simulink model "parametrefarkli"  (R2017b)
settings: Solver=VariableStepAuto  StartTime=0.0  StopTime=10.0  RelTol=1e-3
undefined symbols (not defined in the file or in its folder): Ts_Power
libraries: powerlib x65, powerlib_extras x60, powerlib_meascontrol x5, simulink x3, re_lib x3
(part 1 of 3)
settings Model: Creator=ongun  LastModifiedBy=ongun

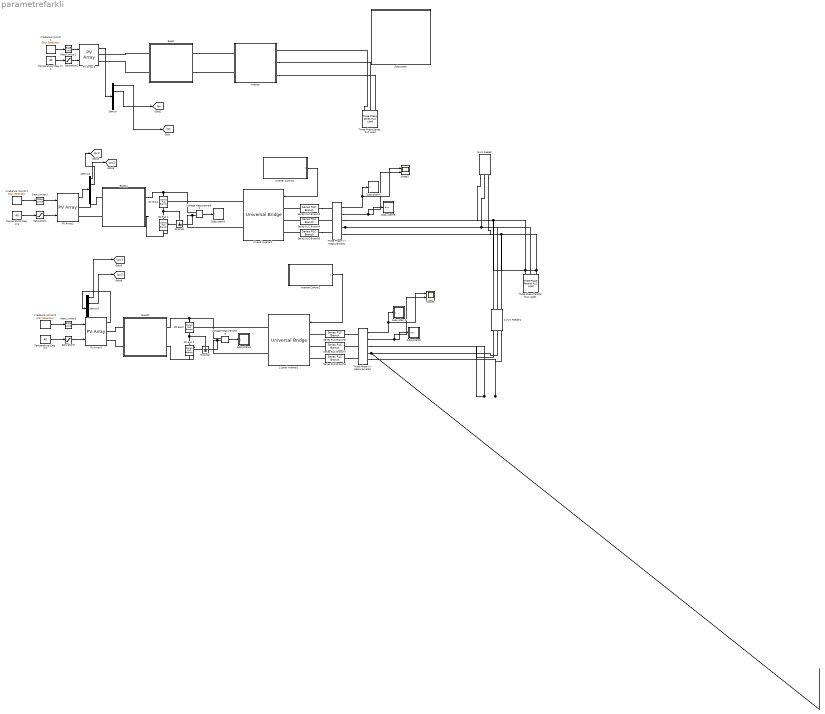
== system parametrefarkli ==
  11-km Feeder1 : powerlib/Elements/Distributed Parameters Line  Phases=3  Frequency=50  Resistance=[0.1153 0.413]  Inductance=[1.05e-3 3.32e-3]  Capacitance=[11.33e-009 5.01e-009]  Length=3  x1=[0 0 0;0 0 0;1.5707963267949 1.5707963267949 1.5707963267949]  x2=[0 0 0;0 0 0;1.5707963267949 1.5707963267949 1.5707963267949]  x3=[0 0 0;0 0 0;1.5707963267949 1.5707963267949 1.5707963267949]  x4=[0 0 0;0 0 0;1.5707963267949 1.5707963267949 1.5707963267949]  x5=1.22351460963897e-05  V1=[0 0 0;0 0 0;1.571 1.571 1.571]  V2=[0 0 0;0 0 0;1.571 1.571 1.571]  I1=[0 0 0;0 0 0;1.571 1.571 1.571]  I2=[0 0 0;0 0 0;1.571 1.571 1.571]  nHarmo=1  Measurements=None
      settings: SourceProductName=Simscape Power Systems
  2 Level Inverter1 : powerlib/Power Electronics/Universal Bridge  Arms=3  SnubberResistance=1e5  SnubberCapacitance=inf  Device=IGBT / Diodes  Ron=1e-3  Lon=0  ForwardVoltages="[  0  0  ]"  ForwardVoltage=0  GTOparameters=[ 10e-6 , 20e-6 ]  IGBTparameters=[ 1e-6 , 2e-6 ]  Measurements=UAB UBC UCA UDC voltages  Measurements_2=None  converterType=Rectifier
  2 Level Inverter2 : powerlib/Power Electronics/Universal Bridge  Arms=3  SnubberResistance=1e5  SnubberCapacitance=inf  Device=IGBT / Diodes  Ron=1e-3  Lon=0  ForwardVoltages="[  0  0  ]"  ForwardVoltage=0  GTOparameters=[ 10e-6 , 20e-6 ]  IGBTparameters=[ 1e-6 , 2e-6 ]  Measurements=UAB UBC UCA UDC voltages  Measurements_2=None  converterType=Rectifier
  8-km Feeder : powerlib/Elements/Distributed Parameters Line  Phases=3  Frequency=50  Resistance=[0.1153 0.413]  Inductance=[1.05e-3 3.32e-3]  Capacitance=[11.33e-009 5.01e-009]  Length=100  x1=[0 0 0;0 0 0;1.5707963267949 1.5707963267949 1.5707963267949]  x2=[0 0 0;0 0 0;1.5707963267949 1.5707963267949 1.5707963267949]  x3=[0 0 0;0 0 0;1.5707963267949 1.5707963267949 1.5707963267949]  x4=[0 0 0;0 0 0;1.5707963267949 1.5707963267949 1.5707963267949]  x5=0.00040783820321299  V1=[0 0 0;0 0 0;1.571 1.571 1.571]  V2=[0 0 0;0 0 0;1.571 1.571 1.571]  I1=[0 0 0;0 0 0;1.571 1.571 1.571]  I2=[0 0 0;0 0 0;1.571 1.571 1.571]  nHarmo=1  Measurements=None
      settings: SourceProductName=Simscape Power Systems
  Boost : Subsystem
      mask Display: disp('Boost Converter')
  Boost1 : Subsystem
      mask Display: disp('Boost Converter')
  Boost2 : Subsystem
      mask Display: disp('Boost Converter')
  DC Bus 1 : powerlib/Elements/Series RLC Branch  LConnTagsString=__new0  RConnTagsString=__new0  BranchType=C  Resistance=1  Inductance=5e-03  SetiL0=off  InitialCurrent=0  Capacitance=10e-3/2  Setx0=off  InitialVoltage=1000/2  Measurements=None
  DC Bus 2 : powerlib/Elements/Series RLC Branch  LConnTagsString=__new0  RConnTagsString=__new0  BranchType=C  Resistance=1  Inductance=5e-03  SetiL0=off  InitialCurrent=0  Capacitance=10e-3/2  Setx0=off  InitialVoltage=1000/2  Measurements=None
  DC Bus1 : powerlib/Elements/Series RLC Branch  LConnTagsString=__new0  RConnTagsString=__new0  BranchType=C  Resistance=1  Inductance=5e-03  SetiL0=off  InitialCurrent=0  Capacitance=10e-3/2  Setx0=off  InitialVoltage=1000/2  Measurements=None
  DC Bus2 : powerlib/Elements/Series RLC Branch  LConnTagsString=__new0  RConnTagsString=__new0  BranchType=C  Resistance=1  Inductance=5e-03  SetiL0=off  InitialCurrent=0  Capacitance=10e-3/2  Setx0=off  InitialVoltage=1000/2  Measurements=None
  Demux : Demux  Outputs=5
  Demux2 : Demux  Outputs=5
  Demux3 : Demux  Outputs=5
  Ground1 : powerlib/Elements/Ground  LConnTagsString=a
  Ground2 : powerlib/Elements/Ground  LConnTagsString=a
  Inverter : Subsystem
      mask Display: disp('DC/AC Inverter')
  Inverter Control1 : Subsystem
  Inverter Control2 : Subsystem
  Irradiance (W/m2) 1 : powerlib_meascontrol/Pulse & Signal Generators/Stair Generator  t=[0, 0.5, 2.3]  e=[1,0.05, 1.0]*1000  Ts=Ts_Power
      settings: SourceProductName=Simscape Power Systems
  Irradiance (W/m2)1 : powerlib_meascontrol/Pulse & Signal Generators/Stair Generator  t=[0, 0.4, 1.0]  e=[1, 0.2, 1]*1000  Ts=5e-5
      settings: SourceProductName=Simscape Power Systems
  Irradiance (W/m2)2 : powerlib_meascontrol/Pulse & Signal Generators/Stair Generator  t=[0, 0.4, 1.0]  e=[1, 0.2, 1]*1000  Ts=5e-5
      settings: SourceProductName=Simscape Power Systems
  PV Array 1 : re_lib/Solar/PV Array  Npar=64  Nser=5  PlotType=array @ 1000 W/m2 & specified temperatures  S_vec="[ 1000  500  100 ]"  Temp_C_vec="[ 45 25  ]"  ModuleName=SunPower SPR-315E-WHT-D  PlotWhenSelected=off  Pm=315.072  Ncell=96  Voc=64.6  Isc=6.14  Vm=54.7  Im=5.76  beta_Voc_pc=-0.27269  alpha_Isc_pc=0.061694  beta_Voc=-0.17616  alpha_Isc=0.003788  IL=6.1461  I0=6.5043e-12  nI=0.9507  Rsh=430.0559  Rs=0.43042  BAL=off  Tc=1e-6  Tfilter=5e-5
  PV Array2 : re_lib/Solar/PV Array  Npar=88  Nser=7  PlotType=array @ 1000 W/m2 & specified temperatures  S_vec="[ 1000  500  100 ]"  Temp_C_vec="[ 45 25  ]"  ModuleName=SunPower SPR-415E-WHT-D  PlotWhenSelected=off  Pm=414.801  Ncell=128  Voc=85.3  Isc=6.09  Vm=72.9  Im=5.69  beta_Voc_pc=-0.229  alpha_Isc_pc=0.030706  beta_Voc=-0.19534  alpha_Isc=0.00187  IL=6.0978  I0=7.1712e-13  nI=0.87223  Rsh=419.7813  Rs=0.5371  BAL=on  Tc=1e-6  Tfilter=5e-5
      settings: AttributesFormatString=|
      | %<ModuleName>
      | %<Nser>-module string
      | %<Npar> parallel strings
  PV Array3 : re_lib/Solar/PV Array  Npar=88  Nser=7  PlotType=array @ 1000 W/m2 & specified temperatures  S_vec="[ 1000  500  100 ]"  Temp_C_vec="[ 45 25  ]"  ModuleName=SunPower SPR-415E-WHT-D  PlotWhenSelected=off  Pm=414.801  Ncell=128  Voc=85.3  Isc=6.09  Vm=72.9  Im=5.69  beta_Voc_pc=-0.229  alpha_Isc_pc=0.030706  beta_Voc=-0.19534  alpha_Isc=0.00187  IL=6.0978  I0=7.1712e-13  nI=0.87223  Rsh=419.7813  Rs=0.5371  BAL=on  Tc=1e-6  Tfilter=5e-5
      settings: AttributesFormatString=|
      | %<ModuleName>
      | %<Nser>-module string
      | %<Npar> parallel strings
  Rate Limiter1 : RateLimiter  RisingSlewLimit=6000  FallingSlewLimit=-6000  SampleTimeMode=inherited  InitialCondition=1000
  Rate Limiter2 : RateLimiter  RisingSlewLimit=8000  FallingSlewLimit=-8000  SampleTimeMode=inherited  InitialCondition=1000
  Rate Limiter3 : RateLimiter  RisingSlewLimit=6000  FallingSlewLimit=-6000  SampleTimeMode=inherited  InitialCondition=1000
  Saturation1 : Saturate  UpperLimit=55  LowerLimit=5
  Saturation2 : Saturate  UpperLimit=55  LowerLimit=5
  Saturation3 : Saturate  UpperLimit=55  LowerLimit=5
  Scope1 : Scope  NumInputPorts=2
  Scope2 : Scope  NumInputPorts=2
  Series RLC Branch{4..9} (6 alike) : powerlib/Elements/Series RLC Branch  LConnTagsString=__new0  RConnTagsString=__new0  BranchType=RL  Resistance=0.1  Inductance=30e-3  SetiL0=off  InitialCurrent=0  Capacitance=1e-6  Setx0=off  InitialVoltage=0  Measurements=Branch voltage
  Subsystem : Subsystem
      mask Display: disp('Measurements')
  Subsystem4 : Subsystem
  Subsystem5 : Subsystem
  Subsystem6 : Subsystem
  Subsystem7 : Subsystem
  Subsystem8 : Subsystem
  Subsystem9 : Subsystem
  Temperature (Deg. C) 1 : Constant  Value=40
  Temperature (Deg. C)1 : Constant  Value=40
  Temperature (Deg. C)2 : Constant  Value=40
  Three-Phase Parallel RLC Load1 : powerlib/Elements/Three-Phase Parallel RLC Load  LConnTagsString=A|B|C  Configuration=Y (grounded)  NominalVoltage=(25000)*1  Vabc=[1e3 1e3 1e3]  Vabcp=[1e3 1e3 1e3]  NominalFrequency=60  UnbalancedPower=off  ActivePower=100e3  InductivePower=0  CapacitivePower=0  Pabc=[10e3 9e3 11e3]  QLabc=[100 90 110]  QCabc=[100 90 110]  Pabcp=[10e3 9e3 11e3]  QLabcp=[100 90 110]  QCabcp=[100 90 110]  Measurements=None  LoadType=constant PQ
  Three-Phase Series RLC Load : powerlib/Elements/Three-Phase Series RLC Load  LConnTagsString=A|B|C  Configuration=Y (grounded)  NominalVoltage=1000  Vabc=[1e3 1e3 1e3]  Vabcp=[1e3 1e3 1e3]  NominalFrequency=60  UnbalancedPower=off  ActivePower=10e3  InductivePower=100  CapacitivePower=100  Pabc=[10e3 9e3 11e3]  QLabc=[100 90 110]  QCabc=[100 90 110]  Pabcp=[10e3 9e3 11e3]  QLabcp=[100 90 110]  QCabcp=[100 90 110]  Measurements=None  LoadType=constant Z
  Three-Phase V-I Measurement1 : powerlib/Measurements/Three-Phase V-I Measurement  VoltageMeasurement=phase-to-ground  SetLabelV=off  LabelV=Vabc  Vpu=off  VpuLL=off  CurrentMeasurement=yes  SetLabelI=off  LabelI=Iabc  Ipu=off  Pbase=100e6  Vbase=500e3  OutputType=Complex  PhasorSimulation=off  PSBequivalent=0
  Three-Phase V-I Measurement2 : powerlib/Measurements/Three-Phase V-I Measurement  VoltageMeasurement=phase-to-ground  SetLabelV=off  LabelV=Vabc  Vpu=off  VpuLL=off  CurrentMeasurement=yes  SetLabelI=off  LabelI=Iabc  Ipu=off  Pbase=100e6  Vbase=500e3  OutputType=Complex  PhasorSimulation=off  PSBequivalent=0
  Voltage Measurement2 : powerlib/Measurements/Voltage Measurement  PhasorSimulation=off  OutputType=Complex  PSBequivalent=0
  Voltage Measurement3 : powerlib/Measurements/Voltage Measurement  PhasorSimulation=off  OutputType=Complex  PSBequivalent=0
  tag scope: Ipv2=global, Ipv3=global, Ipv=global, Vpv2=global, Vpv3=global, Vpv=global
  wires:
  PV Array 1/1 -> Demux/1
  Demux/1 -> [Vpv]
  Demux/2 -> [Ipv]
  Rate Limiter2/1 -> PV Array 1/1
  Temperature (Deg. C) 1/1 -> Saturation2/1
  Saturation2/1 -> PV Array 1/2
  Irradiance (W/m2) 1/1 -> Rate Limiter2/1
  Demux3/1 -> [Vpv3]
  Demux3/2 -> [Ipv3]
  Three-Phase V-I Measurement2/1 -> Scope2/1, Subsystem7/1(Vabc)
  Saturation3/1 -> PV Array3/2
  Inverter Control2/1(S) -> 2 Level Inverter2/1
  Voltage Measurement3/1 -> Subsystem8/1(Vdcinv)
  Three-Phase V-I Measurement2/2 -> Scope2/2, Subsystem9/1(Iabc)
  Temperature (Deg. C)1/1 -> Saturation1/1
  Three-Phase V-I Measurement1/2 -> Scope1/2, Subsystem6/1(Iabc)
  Rate Limiter1/1 -> PV Array2/1
  Voltage Measurement2/1 -> Subsystem5/1(Vdcinv)
  Inverter Control1/1(S) -> 2 Level Inverter1/1
  Three-Phase V-I Measurement1/1 -> Scope1/1, Subsystem4/1(Vabc)
  PV Array2/1 -> Demux2/1
  Irradiance (W/m2)2/1 -> Rate Limiter3/1
  Rate Limiter3/1 -> PV Array3/1
  Saturation1/1 -> PV Array2/2
  PV Array3/1 -> Demux3/1
  Temperature (Deg. C)2/1 -> Saturation3/1
  Irradiance (W/m2)1/1 -> Rate Limiter1/1
  Demux2/2 -> [Ipv2]
  Demux2/1 -> [Vpv2]
  connections:
  Boost/LConn2 -- PV Array 1/RConn2
  Boost/RConn2 -- Inverter/RConn2
  Inverter/LConn2 -- Three-Phase Series RLC Load/LConn2
  Inverter/LConn3 -- Three-Phase Series RLC Load/LConn3
  Boost/LConn1 -- PV Array 1/RConn1
  Boost/RConn1 -- Inverter/RConn1
  Three-Phase Series RLC Load/LConn1 -- Inverter/LConn1
  Three-Phase V-I Measurement2/RConn3 -- 11-km Feeder1/RConn3
  Voltage Measurement2/LConn2 -- Boost1/RConn2 -- DC Bus 1/RConn1 -- 2 Level Inverter1/RConn2
  DC Bus2/LConn1 -- Boost2/RConn1 -- 2 Level Inverter2/RConn1 -- Voltage Measurement3/LConn1
  DC Bus1/RConn1 -- Ground1/LConn1 -- DC Bus 1/LConn1
  Three-Phase Parallel RLC Load1/LConn3 -- Three-Phase V-I Measurement1/RConn3 -- 8-km Feeder/RConn3 -- 11-km Feeder1/LConn3
  DC Bus2/RConn1 -- Ground2/LConn1 -- DC Bus 2/LConn1
  Three-Phase V-I Measurement2/RConn1 -- 11-km Feeder1/RConn1
  Voltage Measurement3/LConn2 -- Boost2/RConn2 -- DC Bus 2/RConn1 -- 2 Level Inverter2/RConn2
  Three-Phase Parallel RLC Load1/LConn1 -- Three-Phase V-I Measurement1/RConn1 -- 8-km Feeder/RConn1 -- 11-km Feeder1/LConn1
  Three-Phase V-I Measurement1/RConn2 -- 8-km Feeder/RConn2 -- Three-Phase Parallel RLC Load1/LConn2 -- 11-km Feeder1/LConn2
  Three-Phase V-I Measurement2/RConn2 -- 11-km Feeder1/RConn2
  DC Bus1/LConn1 -- Boost1/RConn1 -- 2 Level Inverter1/RConn1 -- Voltage Measurement2/LConn1
  Boost2/LConn2 -- PV Array3/RConn2
  Boost2/LConn1 -- PV Array3/RConn1
  Boost1/LConn2 -- PV Array2/RConn2
  Series RLC Branch6/RConn1 -- Three-Phase V-I Measurement1/LConn3
  Boost1/LConn1 -- PV Array2/RConn1
  Three-Phase V-I Measurement2/LConn2 -- Series RLC Branch7/RConn1
  Series RLC Branch9/LConn1 -- 2 Level Inverter2/LConn3
  Series RLC Branch4/LConn1 -- 2 Level Inverter1/LConn2
  Series RLC Branch8/LConn1 -- 2 Level Inverter2/LConn1
  Series RLC Branch7/LConn1 -- 2 Level Inverter2/LConn2
  Series RLC Branch5/LConn1 -- 2 Level Inverter1/LConn1
  Series RLC Branch8/RConn1 -- Three-Phase V-I Measurement2/LConn1
  Series RLC Branch5/RConn1 -- Three-Phase V-I Measurement1/LConn1
  Three-Phase V-I Measurement1/LConn2 -- Series RLC Branch4/RConn1
  Series RLC Branch9/RConn1 -- Three-Phase V-I Measurement2/LConn3
  Series RLC Branch6/LConn1 -- 2 Level Inverter1/LConn3

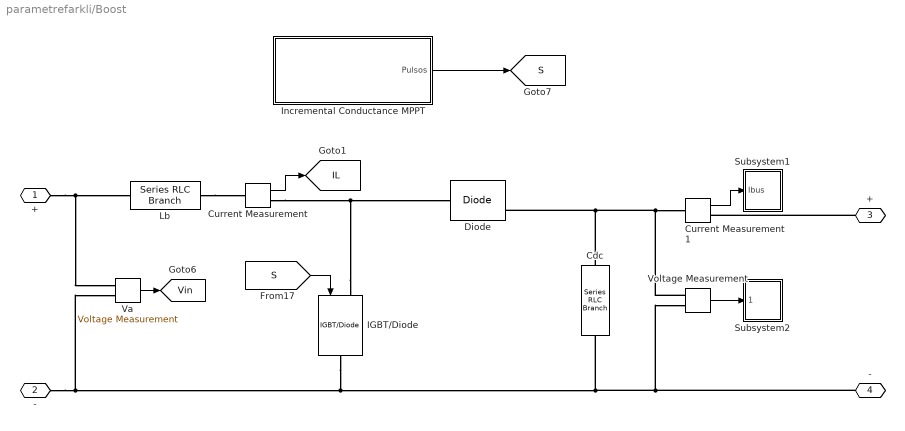
== system parametrefarkli/Boost ==
  Cdc : powerlib/Elements/Series RLC Branch  LConnTagsString=__new0  RConnTagsString=__new0  BranchType=C  Resistance=1  Inductance=1e-3  SetiL0=off  InitialCurrent=0  Capacitance=1200e-6  Setx0=off  InitialVoltage=400  Measurements=None
  Current Measurement : powerlib/Measurements/Current Measurement  PhasorSimulation=off  OutputType=Complex  PSBequivalent=0
  Current Measurement1 : powerlib/Measurements/Current Measurement  PhasorSimulation=off  OutputType=Complex  PSBequivalent=0
  Diode : powerlib/Power Electronics/Diode  Ron=0.001  Lon=0  Vf=0.8  IC=0  UseSnubber=off  Rs=500  Cs=250e-9  Measurements=on
  IGBT/Diode : powerlib/Power Electronics/IGBT//Diode  Ron=1e-3  Rs=1e5  Cs=inf  Measurements=off
  Incremental Conductance MPPT : Subsystem
  Lb : powerlib/Elements/Series RLC Branch  LConnTagsString=__new0  RConnTagsString=__new0  BranchType=L  Resistance=1  Inductance=880e-6  SetiL0=off  InitialCurrent=0  Capacitance=1e-6  Setx0=off  InitialVoltage=0  Measurements=None
  Subsystem1 : Subsystem
  Subsystem2 : Subsystem
  Va : powerlib/Measurements/Voltage Measurement  PhasorSimulation=off  OutputType=Complex  PSBequivalent=0
  Voltage Measurement : powerlib/Measurements/Voltage Measurement  PhasorSimulation=off  OutputType=Complex  PSBequivalent=0
  + : PMIOPort  Port=1  Side=Left
  - : PMIOPort  Port=2  Side=Left
  "+ " : PMIOPort  Port=3  Side=Right
  "- " : PMIOPort  Port=4  Side=Right
  tag scope: IL=global, S=global, Vin=global
  wires:
  Current Measurement/1 -> [IL]
  [S] -> IGBT/Diode/1
  Voltage Measurement/1 -> Subsystem2/1(Vbus)
  Current Measurement1/1 -> Subsystem1/1(Ibus)
  Va/1 -> [Vin]
  Incremental Conductance MPPT/1(Pulsos) -> [S]
  connections:
  Voltage Measurement/LConn1 -- Current Measurement1/LConn1 -- Cdc/LConn1 -- Diode/RConn1
  Cdc/RConn1 -- "- "/RConn1 -- Voltage Measurement/LConn2 -- -/RConn1 -- Va/LConn2 -- IGBT/Diode/RConn1
  Lb/RConn1 -- Current Measurement/LConn1
  IGBT/Diode/LConn1 -- Current Measurement/RConn1 -- Diode/LConn1
  +/RConn1 -- Lb/LConn1 -- Va/LConn1
  "+ "/RConn1 -- Current Measurement1/RConn1

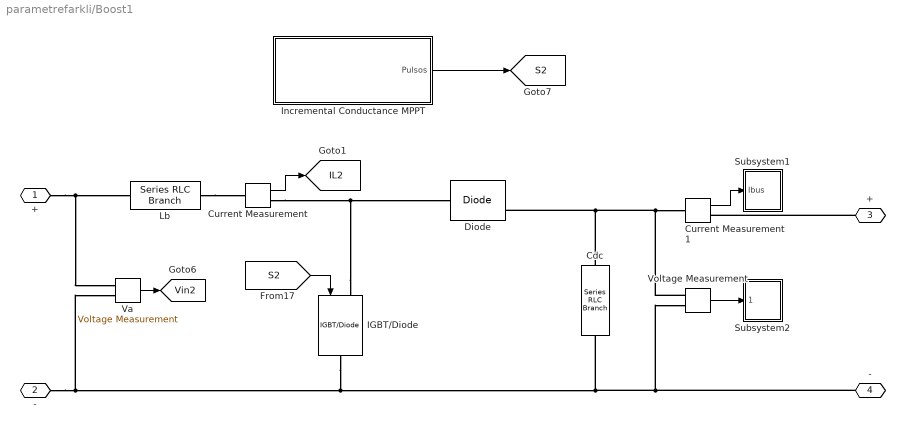
== system parametrefarkli/Boost1 ==
  Cdc : powerlib/Elements/Series RLC Branch  LConnTagsString=__new0  RConnTagsString=__new0  BranchType=C  Resistance=1  Inductance=1e-3  SetiL0=off  InitialCurrent=0  Capacitance=1200e-6  Setx0=off  InitialVoltage=400  Measurements=None
  Current Measurement : powerlib/Measurements/Current Measurement  PhasorSimulation=off  OutputType=Complex  PSBequivalent=0
  Current Measurement1 : powerlib/Measurements/Current Measurement  PhasorSimulation=off  OutputType=Complex  PSBequivalent=0
  Diode : powerlib/Power Electronics/Diode  Ron=0.001  Lon=0  Vf=0.8  IC=0  UseSnubber=off  Rs=500  Cs=250e-9  Measurements=on
  IGBT/Diode : powerlib/Power Electronics/IGBT//Diode  Ron=1e-3  Rs=1e5  Cs=inf  Measurements=off
  Incremental Conductance MPPT : Subsystem
  Lb : powerlib/Elements/Series RLC Branch  LConnTagsString=__new0  RConnTagsString=__new0  BranchType=L  Resistance=1  Inductance=880e-6  SetiL0=off  InitialCurrent=0  Capacitance=1e-6  Setx0=off  InitialVoltage=0  Measurements=None
  Subsystem1 : Subsystem
  Subsystem2 : Subsystem
  Va : powerlib/Measurements/Voltage Measurement  PhasorSimulation=off  OutputType=Complex  PSBequivalent=0
  Voltage Measurement : powerlib/Measurements/Voltage Measurement  PhasorSimulation=off  OutputType=Complex  PSBequivalent=0
  + : PMIOPort  Port=1  Side=Left
  - : PMIOPort  Port=2  Side=Left
  "+ " : PMIOPort  Port=3  Side=Right
  "- " : PMIOPort  Port=4  Side=Right
  tag scope: IL2=global, S2=global, Vin2=global
  wires:
  Current Measurement/1 -> [IL2]
  [S2] -> IGBT/Diode/1
  Voltage Measurement/1 -> Subsystem2/1(Vbus)
  Current Measurement1/1 -> Subsystem1/1(Ibus)
  Va/1 -> [Vin2]
  Incremental Conductance MPPT/1(Pulsos) -> [S2]
  connections:
  Voltage Measurement/LConn1 -- Current Measurement1/LConn1 -- Cdc/LConn1 -- Diode/RConn1
  Cdc/RConn1 -- "- "/RConn1 -- Voltage Measurement/LConn2 -- -/RConn1 -- Va/LConn2 -- IGBT/Diode/RConn1
  Lb/RConn1 -- Current Measurement/LConn1
  IGBT/Diode/LConn1 -- Current Measurement/RConn1 -- Diode/LConn1
  +/RConn1 -- Lb/LConn1 -- Va/LConn1
  "+ "/RConn1 -- Current Measurement1/RConn1

== system parametrefarkli/Boost2 ==
  Cdc : powerlib/Elements/Series RLC Branch  LConnTagsString=__new0  RConnTagsString=__new0  BranchType=C  Resistance=1  Inductance=1e-3  SetiL0=off  InitialCurrent=0  Capacitance=1200e-6  Setx0=off  InitialVoltage=400  Measurements=None
  Current Measurement : powerlib/Measurements/Current Measurement  PhasorSimulation=off  OutputType=Complex  PSBequivalent=0
  Current Measurement1 : powerlib/Measurements/Current Measurement  PhasorSimulation=off  OutputType=Complex  PSBequivalent=0
  Diode : powerlib/Power Electronics/Diode  Ron=0.001  Lon=0  Vf=0.8  IC=0  UseSnubber=off  Rs=500  Cs=250e-9  Measurements=on
  IGBT/Diode : powerlib/Power Electronics/IGBT//Diode  Ron=1e-3  Rs=1e5  Cs=inf  Measurements=off
  Incremental Conductance MPPT : Subsystem
  Lb : powerlib/Elements/Series RLC Branch  LConnTagsString=__new0  RConnTagsString=__new0  BranchType=L  Resistance=1  Inductance=880e-6  SetiL0=off  InitialCurrent=0  Capacitance=1e-6  Setx0=off  InitialVoltage=0  Measurements=None
  Subsystem1 : Subsystem
  Subsystem2 : Subsystem
  Va : powerlib/Measurements/Voltage Measurement  PhasorSimulation=off  OutputType=Complex  PSBequivalent=0
  Voltage Measurement : powerlib/Measurements/Voltage Measurement  PhasorSimulation=off  OutputType=Complex  PSBequivalent=0
  + : PMIOPort  Port=1  Side=Left
  - : PMIOPort  Port=2  Side=Left
  "+ " : PMIOPort  Port=3  Side=Right
  "- " : PMIOPort  Port=4  Side=Right
  tag scope: IL3=global, S3=global, Vin3=global
  wires:
  Incremental Conductance MPPT/1(Pulsos) -> [S3]
  Va/1 -> [Vin3]
  Current Measurement1/1 -> Subsystem1/1(Ibus)
  Voltage Measurement/1 -> Subsystem2/1(Vbus)
  [S3] -> IGBT/Diode/1
  Current Measurement/1 -> [IL3]
  connections:
  "+ "/RConn1 -- Current Measurement1/RConn1
  Va/LConn1 -- Lb/LConn1 -- +/RConn1
  Diode/LConn1 -- Current Measurement/RConn1 -- IGBT/Diode/LConn1
  Lb/RConn1 -- Current Measurement/LConn1
  IGBT/Diode/RConn1 -- Va/LConn2 -- -/RConn1 -- Voltage Measurement/LConn2 -- "- "/RConn1 -- Cdc/RConn1
  Diode/RConn1 -- Cdc/LConn1 -- Current Measurement1/LConn1 -- Voltage Measurement/LConn1

== system parametrefarkli/Inverter ==
  DC / AC Inverter : Subsystem
  "DC BUS " : Subsystem
  Inverter Control : Subsystem
  + : PMIOPort  Port=1  Side=Right
  A : PMIOPort  Port=2  Side=Left
  B : PMIOPort  Port=3  Side=Left
  - : PMIOPort  Port=4  Side=Right
  C : PMIOPort  Port=5  Side=Left
  wires:
  Inverter Control/1(S) -> DC / AC Inverter/1(S)
  connections:
  A/RConn1 -- DC / AC Inverter/LConn1
  B/RConn1 -- DC / AC Inverter/LConn2
  C/RConn1 -- DC / AC Inverter/LConn3
  "DC BUS "/LConn2 -- DC / AC Inverter/RConn2
  "DC BUS "/LConn1 -- DC / AC Inverter/RConn1
  +/RConn1 -- "DC BUS "/RConn1
  -/RConn1 -- "DC BUS "/RConn2

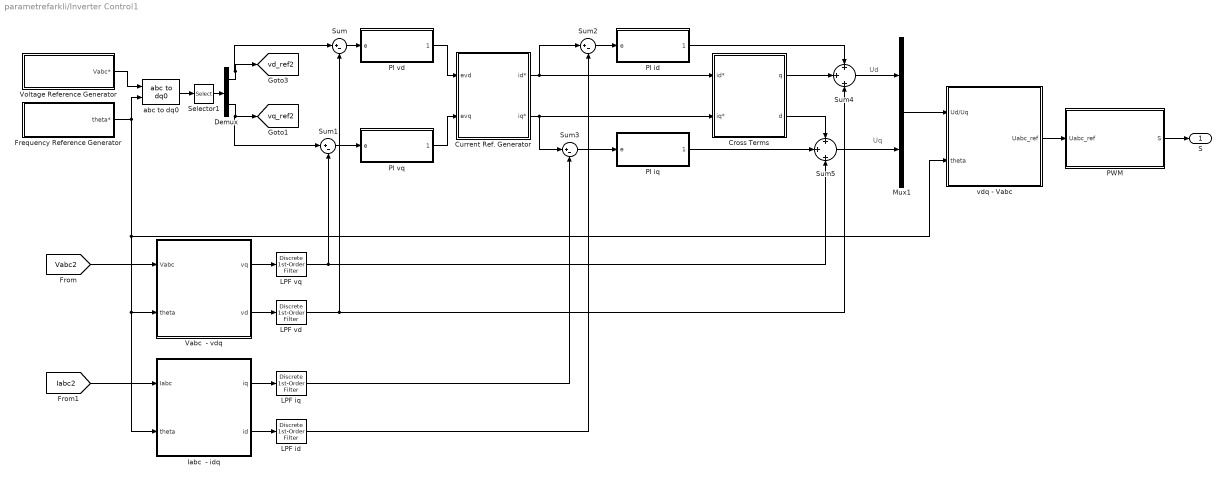
== system parametrefarkli/Inverter Control1 ==
  note: Ud
  note: Uq
  " Voltage Reference Generator" : Subsystem
  Cross Terms : Subsystem
  Current Ref. Generator : Subsystem
  Demux : Demux  Outputs=2
  Frequency Reference Generator : Subsystem
  Iabc  - idq : Subsystem
  LPF id : powerlib_extras/Discrete  Control Blocks/Discrete 1st-Order Filter  FilterType=Lowpass  Tc=1e-3  Ts=5e-6  Initialize=off  Vac_Init=[0.8 -25 60]  Vdc_Init=0  PlotResponse=off  param1=[1 100 0.1]
  LPF iq : powerlib_extras/Discrete  Control Blocks/Discrete 1st-Order Filter  FilterType=Lowpass  Tc=1e-3  Ts=5e-6  Initialize=off  Vac_Init=[0.8 -25 60]  Vdc_Init=0  PlotResponse=off  param1=[1 100 0.1]
  LPF vd : powerlib_extras/Discrete  Control Blocks/Discrete 1st-Order Filter  FilterType=Lowpass  Tc=10e-3  Ts=5e-6  Initialize=off  Vac_Init=[0.8 -25 60]  Vdc_Init=-0.4  PlotResponse=off  param1=[1 100 0.1]
  LPF vq : powerlib_extras/Discrete  Control Blocks/Discrete 1st-Order Filter  FilterType=Lowpass  Tc=10e-3  Ts=5e-6  Initialize=off  Vac_Init=[0.8 -25 60]  Vdc_Init=0  PlotResponse=off  param1=[1 100 0.1]
  Mux1 : Mux  Inputs=2
  PI id : Subsystem
  PI iq : Subsystem
  PI vd : Subsystem
  PI vq : Subsystem
  PWM : Subsystem
  Selector1 : Selector  InputPortWidth=3  IndexOptions=Index vector (dialog)  Indices=[1 2]  OutputSizes=1
  Sum{,1..3} (4 alike) : Sum  Inputs=|+-
  Sum4 : Sum  Inputs=+|+|+
  Sum5 : Sum  Inputs=+|+|+
  Vabc  - vdq : Subsystem
  abc to dq0 : powerlib_meascontrol/Transformations/abc to dq0  Alignment=90 degrees behind phase A axis
  vdq - Vabc : Subsystem
  S : Outport
  tag scope: vd_ref2=global, vq_ref2=global
  wires:
  [Vabc2] -> Vabc  - vdq/1(Vabc)
  [Iabc2] -> Iabc  - idq/1(Iabc)
  Sum2/1 -> PI id/1(e)
  Sum3/1 -> PI iq/1(e)
  Mux1/1 -> vdq - Vabc/1(Ud/Uq)
  vdq - Vabc/1(Uabc_ref) -> PWM/1(Uabc_ref)
  PWM/1(S) -> S/1
  Vabc  - vdq/2(vd) -> LPF vd/1
  Iabc  - idq/1(iq) -> LPF iq/1
  Iabc  - idq/2(id) -> LPF id/1
  LPF vd/1 -> Sum/2, Sum4/3
  LPF vq/1 -> Sum1/2, Sum5/3
  LPF iq/1 -> Sum3/2
  LPF id/1 -> Sum2/2
  Sum/1 -> PI vd/1(e)
  Sum1/1 -> PI vq/1(e)
  Vabc  - vdq/1(vq) -> LPF vq/1
  Demux/1 -> Sum/1, [vd_ref2]
  Demux/2 -> Sum1/1, [vq_ref2]
  " Voltage Reference Generator"/1(Vabc*) -> abc to dq0/1
  Frequency Reference Generator/1(theta*) -> abc to dq0/2, Vabc  - vdq/2(theta), Iabc  - idq/2(theta), vdq - Vabc/2(theta)
  PI vd/1(" ") -> Current Ref. Generator/1(evd)
  PI vq/1(" ") -> Current Ref. Generator/2(evq)
  Current Ref. Generator/2(iq*) -> Sum3/1, Cross Terms/2(iq*)
  Current Ref. Generator/1(id*) -> Sum2/1, Cross Terms/1(id*)
  PI iq/1(" ") -> Sum5/2
  PI id/1(" ") -> Sum4/1
  Cross Terms/1(" q") -> Sum4/2
  Cross Terms/2(" d") -> Sum5/1
  Sum5/1 -> Mux1/2
  Sum4/1 -> Mux1/1
  abc to dq0/1 -> Selector1/1
  Selector1/1 -> Demux/1

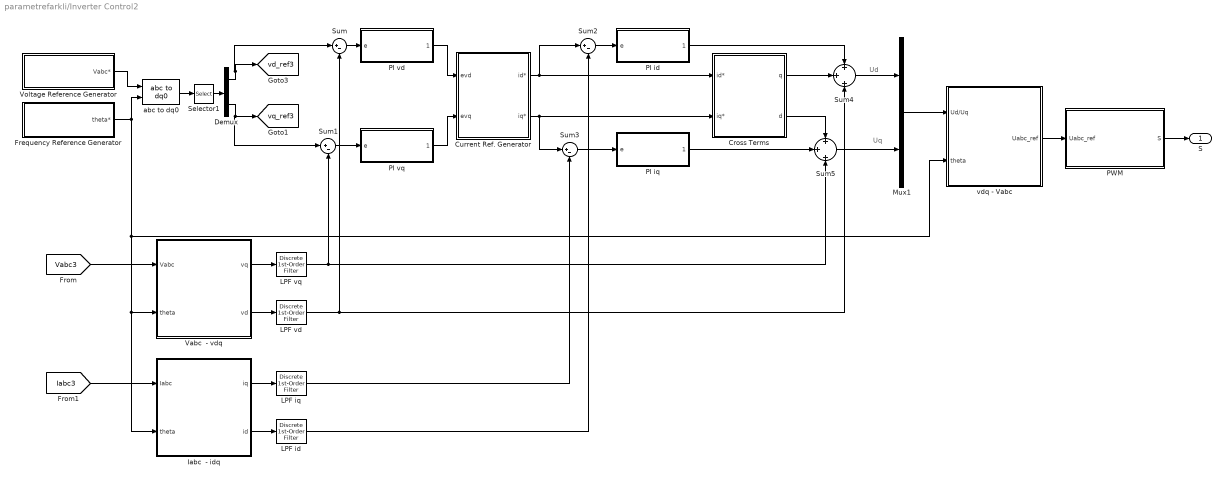
== system parametrefarkli/Inverter Control2 ==
  note: Ud
  note: Uq
  " Voltage Reference Generator" : Subsystem
  Cross Terms : Subsystem
  Current Ref. Generator : Subsystem
  Demux : Demux  Outputs=2
  Frequency Reference Generator : Subsystem
  Iabc  - idq : Subsystem
  LPF id : powerlib_extras/Discrete  Control Blocks/Discrete 1st-Order Filter  FilterType=Lowpass  Tc=1e-3  Ts=5e-6  Initialize=off  Vac_Init=[0.8 -25 60]  Vdc_Init=0  PlotResponse=off  param1=[1 100 0.1]
  LPF iq : powerlib_extras/Discrete  Control Blocks/Discrete 1st-Order Filter  FilterType=Lowpass  Tc=1e-3  Ts=5e-6  Initialize=off  Vac_Init=[0.8 -25 60]  Vdc_Init=0  PlotResponse=off  param1=[1 100 0.1]
  LPF vd : powerlib_extras/Discrete  Control Blocks/Discrete 1st-Order Filter  FilterType=Lowpass  Tc=10e-3  Ts=5e-6  Initialize=off  Vac_Init=[0.8 -25 60]  Vdc_Init=-0.4  PlotResponse=off  param1=[1 100 0.1]
  LPF vq : powerlib_extras/Discrete  Control Blocks/Discrete 1st-Order Filter  FilterType=Lowpass  Tc=10e-3  Ts=5e-6  Initialize=off  Vac_Init=[0.8 -25 60]  Vdc_Init=0  PlotResponse=off  param1=[1 100 0.1]
  Mux1 : Mux  Inputs=2
  PI id : Subsystem
  PI iq : Subsystem
  PI vd : Subsystem
  PI vq : Subsystem
  PWM : Subsystem
  Selector1 : Selector  InputPortWidth=3  IndexOptions=Index vector (dialog)  Indices=[1 2]  OutputSizes=1
  Sum{,1..3} (4 alike) : Sum  Inputs=|+-
  Sum4 : Sum  Inputs=+|+|+
  Sum5 : Sum  Inputs=+|+|+
  Vabc  - vdq : Subsystem
  abc to dq0 : powerlib_meascontrol/Transformations/abc to dq0  Alignment=90 degrees behind phase A axis
  vdq - Vabc : Subsystem
  S : Outport
  tag scope: vd_ref3=global, vq_ref3=global
  wires:
  [Vabc3] -> Vabc  - vdq/1(Vabc)
  [Iabc3] -> Iabc  - idq/1(Iabc)
  Sum2/1 -> PI id/1(e)
  Sum3/1 -> PI iq/1(e)
  Mux1/1 -> vdq - Vabc/1(Ud/Uq)
  vdq - Vabc/1(Uabc_ref) -> PWM/1(Uabc_ref)
  PWM/1(S) -> S/1
  Vabc  - vdq/2(vd) -> LPF vd/1
  Iabc  - idq/1(iq) -> LPF iq/1
  Iabc  - idq/2(id) -> LPF id/1
  LPF vd/1 -> Sum/2, Sum4/3
  LPF vq/1 -> Sum1/2, Sum5/3
  LPF iq/1 -> Sum3/2
  LPF id/1 -> Sum2/2
  Sum/1 -> PI vd/1(e)
  Sum1/1 -> PI vq/1(e)
  Vabc  - vdq/1(vq) -> LPF vq/1
  Demux/1 -> Sum/1, [vd_ref3]
  Demux/2 -> Sum1/1, [vq_ref3]
  " Voltage Reference Generator"/1(Vabc*) -> abc to dq0/1
  Frequency Reference Generator/1(theta*) -> abc to dq0/2, Vabc  - vdq/2(theta), Iabc  - idq/2(theta), vdq - Vabc/2(theta)
  PI vd/1(" ") -> Current Ref. Generator/1(evd)
  PI vq/1(" ") -> Current Ref. Generator/2(evq)
  Current Ref. Generator/2(iq*) -> Sum3/1, Cross Terms/2(iq*)
  Current Ref. Generator/1(id*) -> Sum2/1, Cross Terms/1(id*)
  PI iq/1(" ") -> Sum5/2
  PI id/1(" ") -> Sum4/1
  Cross Terms/1(" q") -> Sum4/2
  Cross Terms/2(" d") -> Sum5/1
  Sum5/1 -> Mux1/2
  Sum4/1 -> Mux1/1
  abc to dq0/1 -> Selector1/1
  Selector1/1 -> Demux/1

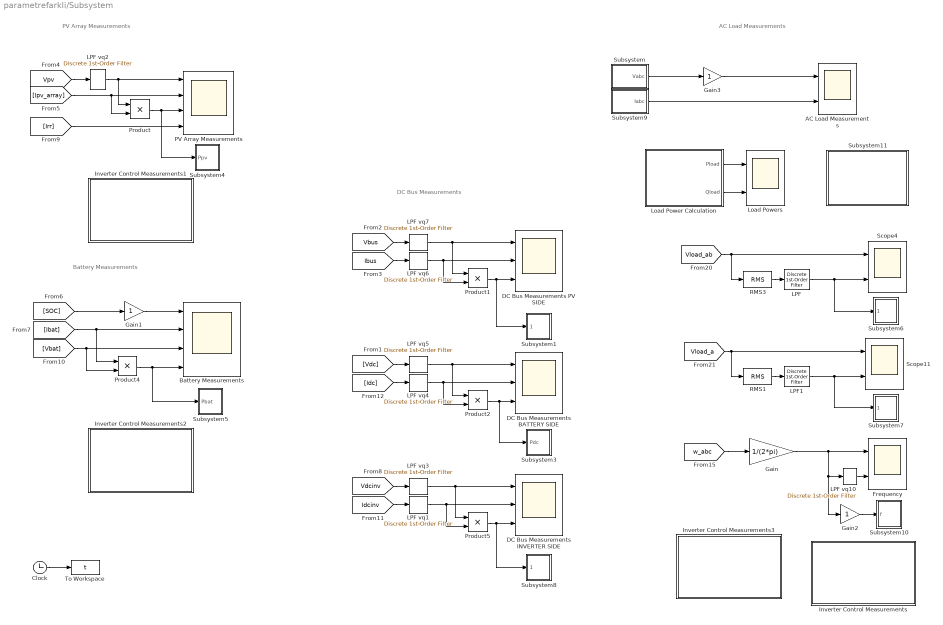
== system parametrefarkli/Subsystem ==
  note: PV Array Measurements
  note: Battery Measurements
  note: DC Bus Measurements
  note: AC Load Measurements
  AC Load Measurements : Scope  NumInputPorts=2
  Battery Measurements : Scope  NumInputPorts=4
  Clock : Clock
  DC Bus Measurements BATTERY SIDE : Scope  NumInputPorts=3
  DC Bus Measurements INVERTER SIDE : Scope  NumInputPorts=3
  DC Bus Measurements PV SIDE : Scope  NumInputPorts=3
  Frequency : Scope  NumInputPorts=2
  Gain : Gain  Gain=1/(2*pi)
  Gain1 : Gain
  Gain2 : Gain
  Gain3 : Gain
  Inverter Control Measurements : Subsystem
      mask Display: disp('Inverter Control')
  Inverter Control Measurements1 : Subsystem
      mask Display: disp('Boost Converter Control')
  Inverter Control Measurements2 : Subsystem
      mask Display: disp('Bidirectional Converter Control')
  Inverter Control Measurements3 : Subsystem
      mask Display: disp('Frequency Measurement')
  LPF : powerlib_extras/Discrete  Control Blocks/Discrete 1st-Order Filter  FilterType=Lowpass  Tc=10e-3  Ts=5e-6  Initialize=off  Vac_Init=[0.8 -25 60]  Vdc_Init=0  PlotResponse=off  param1=[1 100 0.1]
  LPF vq{1..7,10} (8 alike) : powerlib_extras/Discrete  Control Blocks/Discrete 1st-Order Filter  FilterType=Lowpass  Tc=10e-3  Ts=5e-6  Initialize=off  Vac_Init=[0.8 -25 60]  Vdc_Init=0  PlotResponse=off  param1=[1 100 0.1]
  LPF1 : powerlib_extras/Discrete  Control Blocks/Discrete 1st-Order Filter  FilterType=Lowpass  Tc=10e-3  Ts=5e-6  Initialize=off  Vac_Init=[0.8 -25 60]  Vdc_Init=0  PlotResponse=off  param1=[1 100 0.1]
  Load Power Calculation : Subsystem
  Load Powers : Scope  NumInputPorts=2
  PV Array Measurements : Scope  NumInputPorts=4
  Product{,1..2,4..5} (5 alike) : Product  RndMeth=Zero
  RMS1 : powerlib_extras/Measurements/RMS  f1=60
  RMS3 : powerlib_extras/Measurements/RMS  f1=60
  Scope11 : Scope  NumInputPorts=2
  Scope4 : Scope  NumInputPorts=2
  Subsystem : Subsystem
  Subsystem1 : Subsystem
  Subsystem10 : Subsystem
  Subsystem11 : Subsystem
      mask Display: disp('Additional Load Meas.')
  Subsystem3 : Subsystem
  Subsystem4 : Subsystem
  Subsystem5 : Subsystem
  Subsystem6 : Subsystem
  Subsystem7 : Subsystem
  Subsystem8 : Subsystem
  Subsystem9 : Subsystem
  To Workspace : ToWorkspace  VariableName=t  SampleTime=5e-6
  wires:
  Product/1 -> PV Array Measurements/3, Subsystem4/1(Ppv)
  [Vpv] -> LPF vq2/1
  [Ipv_array] -> PV Array Measurements/2, Product/2
  [Irr] -> PV Array Measurements/4
  [SOC] -> Gain1/1
  [Ibat] -> Battery Measurements/2, Product4/1
  [Vbat] -> Battery Measurements/3, Product4/2
  Product4/1 -> Battery Measurements/4, Subsystem5/1(Pbat)
  [Vdc] -> LPF vq5/1
  [Idc] -> LPF vq4/1
  Product2/1 -> DC Bus Measurements BATTERY SIDE/3, Subsystem3/1(Pdc)
  Product1/1 -> DC Bus Measurements PV SIDE/3, Subsystem1/1(Pbus)
  [Vbus] -> LPF vq7/1
  [Ibus] -> LPF vq6/1
  Load Power Calculation/1(Pload) -> Load Powers/1
  Load Power Calculation/2(Qload) -> Load Powers/2
  [Vload_a] -> Scope11/1, RMS1/1
  RMS1/1 -> LPF1/1
  [Vload_ab] -> Scope4/1, RMS3/1
  RMS3/1 -> LPF/1
  LPF/1 -> Scope4/2, Subsystem6/1(Vab_rms)
  LPF1/1 -> Scope11/2, Subsystem7/1(Va_rms)
  Clock/1 -> To Workspace/1
  Product5/1 -> Subsystem8/1(Pdcinv), DC Bus Measurements INVERTER SIDE/3
  [Vdcinv] -> LPF vq3/1
  [Idcinv] -> LPF vq1/1
  LPF vq2/1 -> PV Array Measurements/1, Product/1
  LPF vq1/1 -> DC Bus Measurements INVERTER SIDE/2, Product5/2
  LPF vq3/1 -> DC Bus Measurements INVERTER SIDE/1, Product5/1
  LPF vq4/1 -> Product2/2, DC Bus Measurements BATTERY SIDE/2
  LPF vq5/1 -> Product2/1, DC Bus Measurements BATTERY SIDE/1
  LPF vq6/1 -> DC Bus Measurements PV SIDE/2, Product1/2
  LPF vq7/1 -> DC Bus Measurements PV SIDE/1, Product1/1
  [w_abc] -> Gain/1
  Gain/1 -> Frequency/1, LPF vq10/1, Gain2/1
  LPF vq10/1 -> Frequency/2
  Subsystem9/1(Iabc) -> AC Load Measurements/2
  Subsystem/1(Vabc) -> Gain3/1
  Gain1/1 -> Battery Measurements/1
  Gain2/1 -> Subsystem10/1(f)
  Gain3/1 -> AC Load Measurements/1

== system parametrefarkli/Subsystem4 ==
  Vabc : Inport
  To Workspace1 : ToWorkspace  VariableName=Vabc2  SampleTime=-1
  tag scope: Vabc2=global
  wires:
  Vabc/1 -> To Workspace1/1, [Vabc2]

== system parametrefarkli/Subsystem5 ==
  Vdcinv : Inport
  LPF vq11 : powerlib_extras/Discrete  Control Blocks/Discrete 1st-Order Filter  FilterType=Lowpass  Tc=10e-3  Ts=5e-6  Initialize=off  Vac_Init=[0.8 -25 60]  Vdc_Init=0  PlotResponse=off  param1=[1 100 0.1]
  To Workspace1 : ToWorkspace  VariableName=Vdcinv2  SampleTime=-1
  To Workspace2 : ToWorkspace  VariableName=Vdcinv21  SampleTime=-1
  tag scope: Vdcinv2=global
  wires:
  Vdcinv/1 -> [Vdcinv2], To Workspace1/1, LPF vq11/1
  LPF vq11/1 -> To Workspace2/1

== system parametrefarkli/Subsystem6 ==
  Iabc : Inport
  To Workspace1 : ToWorkspace  VariableName=Iabc2  SampleTime=-1
  tag scope: Iabc2=global
  wires:
  Iabc/1 -> [Iabc2], To Workspace1/1

== system parametrefarkli/Subsystem7 ==
  Vabc : Inport
  To Workspace1 : ToWorkspace  VariableName=Vabc3  SampleTime=-1
  tag scope: Vabc3=global
  wires:
  Vabc/1 -> To Workspace1/1, [Vabc3]

== system parametrefarkli/Subsystem8 ==
  Vdcinv : Inport
  LPF vq11 : powerlib_extras/Discrete  Control Blocks/Discrete 1st-Order Filter  FilterType=Lowpass  Tc=10e-3  Ts=5e-6  Initialize=off  Vac_Init=[0.8 -25 60]  Vdc_Init=0  PlotResponse=off  param1=[1 100 0.1]
  To Workspace1 : ToWorkspace  VariableName=Vdcinv3  SampleTime=-1
  To Workspace2 : ToWorkspace  VariableName=Vdcinv31  SampleTime=-1
  tag scope: Vdcinv3=global
  wires:
  Vdcinv/1 -> [Vdcinv3], To Workspace1/1, LPF vq11/1
  LPF vq11/1 -> To Workspace2/1

== system parametrefarkli/Subsystem9 ==
  Iabc : Inport
  To Workspace1 : ToWorkspace  VariableName=Iabc3  SampleTime=-1
  tag scope: Iabc3=global
  wires:
  Iabc/1 -> [Iabc3], To Workspace1/1

== system parametrefarkli/Boost/Incremental Conductance MPPT ==
  Demux : Demux  Outputs=2
  MPPT IC : MATLAB Function  TreatAsAtomicUnit=on
  Memory{,1..2,4..5} (5 alike) : Memory
  PWM Generator : powerlib_extras/Control  Blocks/PWM Generator  GeneratorMode="1-arm  bridge (2 pulses)"  Fc=10e3  Internal=off  mIndex=0.4  Freq=60  Phase=0
      link override Triangle: rep_seq_t=[0 1/Fc/2 1/Fc]  rep_seq_y=[0 1 0]
  Subsystem1 : Subsystem
  Subsystem2 : Subsystem
  Subsystem3 : Subsystem
  Pulsos : Outport
  wires:
  Memory2/1 -> MPPT IC/4(Vprevious)
  Memory5/1 -> MPPT IC/5(Vref_previous)
  Memory4/1 -> MPPT IC/2(Iprevious)
  Memory1/1 -> MPPT IC/3(Vpv)
  Memory/1 -> MPPT IC/1(Ipv)
  PWM Generator/1 -> Demux/1
  Demux/2 -> Pulsos/1, Subsystem3/1(pulsos)
  MPPT IC/1(delta) -> Subsystem2/1(delta), PWM Generator/1
  MPPT IC/3(Ipv_prev_out) -> Memory4/1
  MPPT IC/4(Vpv_prev_out) -> Memory2/1
  MPPT IC/2(Vref) -> Memory5/1, Subsystem1/1(Vref)
  [Ipv] -> Memory/1
  [Vpv] -> Memory1/1

== system parametrefarkli/Boost/Subsystem1 ==
  Ibus : Inport
  LPF vq11 : powerlib_extras/Discrete  Control Blocks/Discrete 1st-Order Filter  FilterType=Lowpass  Tc=10e-3  Ts=5e-6  Initialize=off  Vac_Init=[0.8 -25 60]  Vdc_Init=0  PlotResponse=off  param1=[1 100 0.1]
  To Workspace1 : ToWorkspace  VariableName=Ibus  SampleTime=-1
  To Workspace2 : ToWorkspace  VariableName=Ibus1  SampleTime=-1
  tag scope: Ibus=global
  wires:
  Ibus/1 -> [Ibus], To Workspace1/1, LPF vq11/1
  LPF vq11/1 -> To Workspace2/1

== system parametrefarkli/Boost/Subsystem2 ==
  Vbus : Inport
  LPF vq11 : powerlib_extras/Discrete  Control Blocks/Discrete 1st-Order Filter  FilterType=Lowpass  Tc=10e-3  Ts=5e-6  Initialize=off  Vac_Init=[0.8 -25 60]  Vdc_Init=0  PlotResponse=off  param1=[1 100 0.1]
  To Workspace1 : ToWorkspace  VariableName=Vbus  SampleTime=-1
  To Workspace2 : ToWorkspace  VariableName=Vbus1  SampleTime=-1
  tag scope: Vbus=global
  wires:
  Vbus/1 -> [Vbus], To Workspace1/1, LPF vq11/1
  LPF vq11/1 -> To Workspace2/1

== system parametrefarkli/Boost1/Incremental Conductance MPPT ==
  Demux : Demux  Outputs=2
  MPPT IC : MATLAB Function  TreatAsAtomicUnit=on
  Memory{,1..2,4..5} (5 alike) : Memory
  PWM Generator : powerlib_extras/Control  Blocks/PWM Generator  GeneratorMode="1-arm  bridge (2 pulses)"  Fc=10e3  Internal=off  mIndex=0.4  Freq=60  Phase=0
      link override Triangle: rep_seq_t=[0 1/Fc/2 1/Fc]  rep_seq_y=[0 1 0]
  Subsystem1 : Subsystem
  Subsystem2 : Subsystem
  Subsystem3 : Subsystem
  Pulsos : Outport
  wires:
  Memory2/1 -> MPPT IC/4(Vprevious)
  Memory5/1 -> MPPT IC/5(Vref_previous)
  Memory4/1 -> MPPT IC/2(Iprevious)
  Memory1/1 -> MPPT IC/3(Vpv)
  Memory/1 -> MPPT IC/1(Ipv)
  PWM Generator/1 -> Demux/1
  Demux/2 -> Pulsos/1, Subsystem3/1(pulsos)
  MPPT IC/1(delta) -> Subsystem2/1(delta), PWM Generator/1
  MPPT IC/3(Ipv_prev_out) -> Memory4/1
  MPPT IC/4(Vpv_prev_out) -> Memory2/1
  MPPT IC/2(Vref) -> Memory5/1, Subsystem1/1(Vref)
  [Ipv2] -> Memory/1
  [Vpv2] -> Memory1/1

== system parametrefarkli/Boost1/Subsystem1 ==
  Ibus : Inport
  LPF vq11 : powerlib_extras/Discrete  Control Blocks/Discrete 1st-Order Filter  FilterType=Lowpass  Tc=10e-3  Ts=5e-6  Initialize=off  Vac_Init=[0.8 -25 60]  Vdc_Init=0  PlotResponse=off  param1=[1 100 0.1]
  To Workspace1 : ToWorkspace  VariableName=Ibus2  SampleTime=-1
  To Workspace2 : ToWorkspace  VariableName=Ibus21  SampleTime=-1
  tag scope: Ibus2=global
  wires:
  Ibus/1 -> [Ibus2], To Workspace1/1, LPF vq11/1
  LPF vq11/1 -> To Workspace2/1

== system parametrefarkli/Boost1/Subsystem2 ==
  Vbus : Inport
  LPF vq11 : powerlib_extras/Discrete  Control Blocks/Discrete 1st-Order Filter  FilterType=Lowpass  Tc=10e-3  Ts=5e-6  Initialize=off  Vac_Init=[0.8 -25 60]  Vdc_Init=0  PlotResponse=off  param1=[1 100 0.1]
  To Workspace1 : ToWorkspace  VariableName=Vbus2  SampleTime=-1
  To Workspace2 : ToWorkspace  VariableName=Vbus21  SampleTime=-1
  tag scope: Vbus2=global
  wires:
  Vbus/1 -> [Vbus2], To Workspace1/1, LPF vq11/1
  LPF vq11/1 -> To Workspace2/1

== system parametrefarkli/Boost2/Incremental Conductance MPPT ==
  Demux : Demux  Outputs=2
  MPPT IC : MATLAB Function  TreatAsAtomicUnit=on
  Memory{,1..2,4..5} (5 alike) : Memory
  PWM Generator : powerlib_extras/Control  Blocks/PWM Generator  GeneratorMode="1-arm  bridge (2 pulses)"  Fc=10e3  Internal=off  mIndex=0.4  Freq=60  Phase=0
      link override Triangle: rep_seq_t=[0 1/Fc/2 1/Fc]  rep_seq_y=[0 1 0]
  Subsystem1 : Subsystem
  Subsystem2 : Subsystem
  Subsystem3 : Subsystem
  Pulsos : Outport
  wires:
  [Vpv3] -> Memory1/1
  [Ipv3] -> Memory/1
  MPPT IC/2(Vref) -> Subsystem1/1(Vref), Memory5/1
  MPPT IC/4(Vpv_prev_out) -> Memory2/1
  MPPT IC/3(Ipv_prev_out) -> Memory4/1
  MPPT IC/1(delta) -> PWM Generator/1, Subsystem2/1(delta)
  Demux/2 -> Subsystem3/1(pulsos), Pulsos/1
  PWM Generator/1 -> Demux/1
  Memory/1 -> MPPT IC/1(Ipv)
  Memory1/1 -> MPPT IC/3(Vpv)
  Memory4/1 -> MPPT IC/2(Iprevious)
  Memory5/1 -> MPPT IC/5(Vref_previous)
  Memory2/1 -> MPPT IC/4(Vprevious)

== system parametrefarkli/Boost2/Subsystem1 ==
  Ibus : Inport
  LPF vq11 : powerlib_extras/Discrete  Control Blocks/Discrete 1st-Order Filter  FilterType=Lowpass  Tc=10e-3  Ts=5e-6  Initialize=off  Vac_Init=[0.8 -25 60]  Vdc_Init=0  PlotResponse=off  param1=[1 100 0.1]
  To Workspace1 : ToWorkspace  VariableName=Ibus3  SampleTime=-1
  To Workspace2 : ToWorkspace  VariableName=Ibus31  SampleTime=-1
  tag scope: Ibus3=global
  wires:
  LPF vq11/1 -> To Workspace2/1
  Ibus/1 -> LPF vq11/1, To Workspace1/1, [Ibus3]

== system parametrefarkli/Boost2/Subsystem2 ==
  Vbus : Inport
  LPF vq11 : powerlib_extras/Discrete  Control Blocks/Discrete 1st-Order Filter  FilterType=Lowpass  Tc=10e-3  Ts=5e-6  Initialize=off  Vac_Init=[0.8 -25 60]  Vdc_Init=0  PlotResponse=off  param1=[1 100 0.1]
  To Workspace1 : ToWorkspace  VariableName=Vbus3  SampleTime=-1
  To Workspace2 : ToWorkspace  VariableName=Vbus31  SampleTime=-1
  tag scope: Vbus3=global
  wires:
  LPF vq11/1 -> To Workspace2/1
  Vbus/1 -> LPF vq11/1, To Workspace1/1, [Vbus3]

== system parametrefarkli/Inverter/DC // AC Inverter ==
  S : Inport
  2 Level Inverter : powerlib/Power Electronics/Universal Bridge  Arms=3  SnubberResistance=1e5  SnubberCapacitance=inf  Device=IGBT / Diodes  Ron=1e-3  Lon=0  ForwardVoltages="[  0  0  ]"  ForwardVoltage=0  GTOparameters=[ 10e-6 , 20e-6 ]  IGBTparameters=[ 1e-6 , 2e-6 ]  Measurements=UAB UBC UCA UDC voltages  Measurements_2=None  converterType=Rectifier
  AC Load Measurements : Subsystem
  Series RLC Branch1 : powerlib/Elements/Series RLC Branch  LConnTagsString=__new0  RConnTagsString=__new0  BranchType=RL  Resistance=0.1  Inductance=30e-3  SetiL0=off  InitialCurrent=0  Capacitance=1e-6  Setx0=off  InitialVoltage=0  Measurements=Branch voltage
  Series RLC Branch2 : powerlib/Elements/Series RLC Branch  LConnTagsString=__new0  RConnTagsString=__new0  BranchType=RL  Resistance=0.1  Inductance=30e-3  SetiL0=off  InitialCurrent=0  Capacitance=1e-6  Setx0=off  InitialVoltage=0  Measurements=Branch voltage
  Series RLC Branch3 : powerlib/Elements/Series RLC Branch  LConnTagsString=__new0  RConnTagsString=__new0  BranchType=RL  Resistance=0.1  Inductance=30e-3  SetiL0=off  InitialCurrent=0  Capacitance=1e-6  Setx0=off  InitialVoltage=0  Measurements=Branch voltage
  + : PMIOPort  Port=1  Side=Right
  A : PMIOPort  Port=2  Side=Left
  B : PMIOPort  Port=3  Side=Left
  - : PMIOPort  Port=4  Side=Right
  C : PMIOPort  Port=5  Side=Left
  wires:
  S/1 -> 2 Level Inverter/1
  connections:
  2 Level Inverter/RConn1 -- +/RConn1
  2 Level Inverter/RConn2 -- -/RConn1
  Series RLC Branch2/LConn1 -- 2 Level Inverter/LConn1
  2 Level Inverter/LConn2 -- Series RLC Branch1/LConn1
  2 Level Inverter/LConn3 -- Series RLC Branch3/LConn1
  Series RLC Branch2/RConn1 -- AC Load Measurements/LConn1
  Series RLC Branch1/RConn1 -- AC Load Measurements/LConn2
  Series RLC Branch3/RConn1 -- AC Load Measurements/LConn3
  AC Load Measurements/RConn1 -- A/RConn1
  AC Load Measurements/RConn2 -- B/RConn1
  AC Load Measurements/RConn3 -- C/RConn1

== system parametrefarkli/Inverter/DC BUS  ==
  Current Measurement1 : powerlib/Measurements/Current Measurement  PhasorSimulation=off  OutputType=Complex  PSBequivalent=0
  DC Bus : powerlib/Elements/Series RLC Branch  LConnTagsString=__new0  RConnTagsString=__new0  BranchType=C  Resistance=1  Inductance=5e-03  SetiL0=off  InitialCurrent=0  Capacitance=10e-3/2  Setx0=off  InitialVoltage=1000/2  Measurements=None
  "DC Bus " : powerlib/Elements/Series RLC Branch  LConnTagsString=__new0  RConnTagsString=__new0  BranchType=C  Resistance=1  Inductance=5e-03  SetiL0=off  InitialCurrent=0  Capacitance=10e-3/2  Setx0=off  InitialVoltage=1000/2  Measurements=None
  Ground : powerlib/Elements/Ground  LConnTagsString=a
  Subsystem1 : Subsystem
  Subsystem2 : Subsystem
  Voltage Measurement1 : powerlib/Measurements/Voltage Measurement  PhasorSimulation=off  OutputType=Complex  PSBequivalent=0
  "+ " : PMIOPort  Port=1  Side=Left
  "- " : PMIOPort  Port=2  Side=Left
  "+  " : PMIOPort  Port=3  Side=Right
  "-  " : PMIOPort  Port=4  Side=Right
  wires:
  Voltage Measurement1/1 -> Subsystem2/1(Vdcinv)
  Current Measurement1/1 -> Subsystem1/1(Idcinv)
  connections:
  DC Bus/LConn1 -- "+  "/RConn1 -- Voltage Measurement1/LConn1 -- Current Measurement1/LConn1
  "DC Bus "/LConn1 -- DC Bus/RConn1 -- Ground/LConn1
  "DC Bus "/RConn1 -- "-  "/RConn1 -- "- "/RConn1 -- Voltage Measurement1/LConn2
  Current Measurement1/RConn1 -- "+ "/RConn1

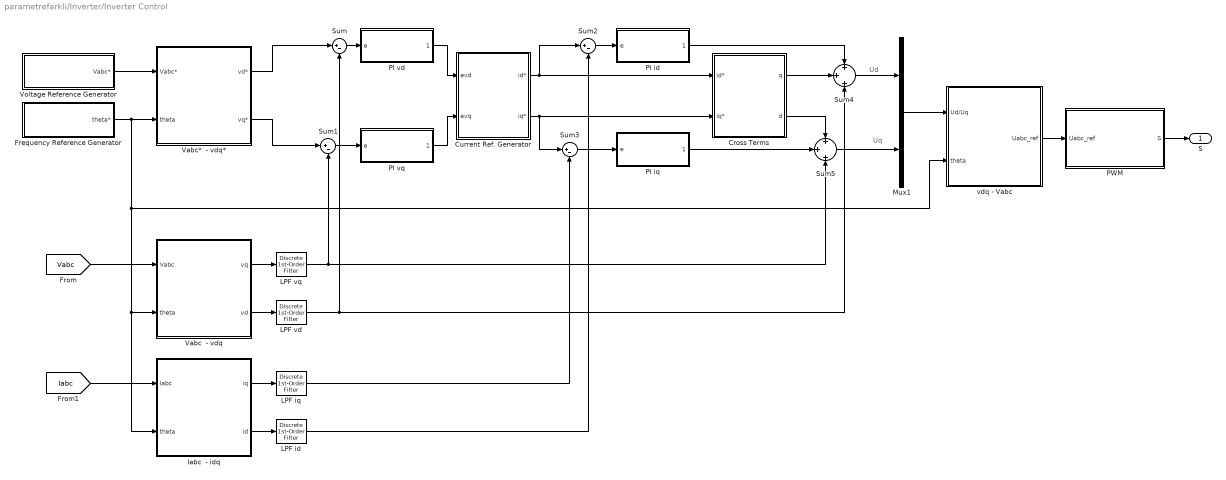
== system parametrefarkli/Inverter/Inverter Control ==
  note: Ud
  note: Uq
  " Voltage Reference Generator" : Subsystem
  Cross Terms : Subsystem
  Current Ref. Generator : Subsystem
  Frequency Reference Generator : Subsystem
  Iabc  - idq : Subsystem
  LPF id : powerlib_extras/Discrete  Control Blocks/Discrete 1st-Order Filter  FilterType=Lowpass  Tc=1e-3  Ts=5e-6  Initialize=off  Vac_Init=[0.8 -25 60]  Vdc_Init=0  PlotResponse=off  param1=[1 100 0.1]
  LPF iq : powerlib_extras/Discrete  Control Blocks/Discrete 1st-Order Filter  FilterType=Lowpass  Tc=1e-3  Ts=5e-6  Initialize=off  Vac_Init=[0.8 -25 60]  Vdc_Init=0  PlotResponse=off  param1=[1 100 0.1]
  LPF vd : powerlib_extras/Discrete  Control Blocks/Discrete 1st-Order Filter  FilterType=Lowpass  Tc=10e-3  Ts=5e-6  Initialize=off  Vac_Init=[0.8 -25 60]  Vdc_Init=-0.4  PlotResponse=off  param1=[1 100 0.1]
  LPF vq : powerlib_extras/Discrete  Control Blocks/Discrete 1st-Order Filter  FilterType=Lowpass  Tc=10e-3  Ts=5e-6  Initialize=off  Vac_Init=[0.8 -25 60]  Vdc_Init=0  PlotResponse=off  param1=[1 100 0.1]
  Mux1 : Mux  Inputs=2
  PI id : Subsystem
  PI iq : Subsystem
  PI vd : Subsystem
  PI vq : Subsystem
  PWM : Subsystem
  Sum{,1..3} (4 alike) : Sum  Inputs=|+-
  Sum4 : Sum  Inputs=+|+|+
  Sum5 : Sum  Inputs=+|+|+
  Vabc  - vdq : Subsystem
  Vabc*  - vdq* : Subsystem
  vdq - Vabc : Subsystem
  S : Outport
  wires:
  [Vabc] -> Vabc  - vdq/1(Vabc)
  [Iabc] -> Iabc  - idq/1(Iabc)
  Sum2/1 -> PI id/1(e)
  Sum3/1 -> PI iq/1(e)
  Mux1/1 -> vdq - Vabc/1(Ud/Uq)
  vdq - Vabc/1(Uabc_ref) -> PWM/1(Uabc_ref)
  PWM/1(S) -> S/1
  Vabc  - vdq/2(vd) -> LPF vd/1
  Iabc  - idq/1(iq) -> LPF iq/1
  Iabc  - idq/2(id) -> LPF id/1
  LPF vd/1 -> Sum/2, Sum4/3
  LPF vq/1 -> Sum1/2, Sum5/3
  LPF iq/1 -> Sum3/2
  LPF id/1 -> Sum2/2
  Sum/1 -> PI vd/1(e)
  Sum1/1 -> PI vq/1(e)
  Vabc  - vdq/1(vq) -> LPF vq/1
  Vabc*  - vdq*/1(vd*) -> Sum/1
  Vabc*  - vdq*/2(vq*) -> Sum1/1
  " Voltage Reference Generator"/1(Vabc*) -> Vabc*  - vdq*/1(Vabc*)
  Frequency Reference Generator/1(theta*) -> Vabc*  - vdq*/2(theta), Vabc  - vdq/2(theta), Iabc  - idq/2(theta), vdq - Vabc/2(theta)
  PI vd/1(" ") -> Current Ref. Generator/1(evd)
  PI vq/1(" ") -> Current Ref. Generator/2(evq)
  Current Ref. Generator/2(iq*) -> Sum3/1, Cross Terms/2(iq*)
  Current Ref. Generator/1(id*) -> Sum2/1, Cross Terms/1(id*)
  PI iq/1(" ") -> Sum5/2
  PI id/1(" ") -> Sum4/1
  Cross Terms/1(" q") -> Sum4/2
  Cross Terms/2(" d") -> Sum5/1
  Sum5/1 -> Mux1/2
  Sum4/1 -> Mux1/1

== system parametrefarkli/Inverter Control1/ Voltage Reference Generator ==
  Mux4 : Mux  Inputs=3
  Phase A reference : Sin  Amplitude=400*sqrt(2)/sqrt(3)  Frequency=2*pi*50  SampleTime=0
  Phase B reference : Sin  Amplitude=400*sqrt(2)/sqrt(3)  Frequency=2*pi*50  Phase=-2*pi/3  SampleTime=0
  Phase C reference : Sin  Amplitude=400*sqrt(2)/sqrt(3)  Frequency=2*pi*50  Phase=2*pi/3  SampleTime=0
  Product : Product  RndMeth=Zero
  Ramp : simulink/Sources/Ramp  slope=1/0.3  start=0  X0=0
  Saturation : Saturate  UpperLimit=1  LowerLimit=0
  Vabc* : Outport
  tag scope: Vabc_ref2=global
  wires:
  Phase B reference/1 -> Mux4/2
  Phase A reference/1 -> Mux4/1
  Phase C reference/1 -> Mux4/3
  Ramp/1 -> Saturation/1
  Saturation/1 -> Product/2
  Mux4/1 -> Vabc*/1, [Vabc_ref2]

== system parametrefarkli/Inverter Control1/Cross Terms ==
  id* : Inport
  iq* : Inport  Port=2
  Gain1 : Gain  Gain=-2*pi*50*3e-3
  Gain2 : Gain  Gain=2*pi*50*3e-3
  " q" : Outport
  " d" : Outport  Port=2
  wires:
  id*/1 -> Gain1/1
  iq*/1 -> Gain2/1
  Gain1/1 -> " d"/1
  Gain2/1 -> " q"/1

== system parametrefarkli/Inverter Control1/Current Ref. Generator ==
  note: evd
  note: evq
  evd : Inport
  evq : Inport  Port=2
  Divide : Product  Inputs=*/
  Divide1 : Product  Inputs=/*
  Scope24 : Scope
  Sum1 : Sum  Inputs=-+|
  Sum3 : Sum  Inputs=|++
  Zd : Gain  Gain=0.4559
  Zd1 : Gain  Gain=0.4559
  Zd^2+Zq^2 : Constant  Value=0.4559^2+0.1824^2
  Zq : Gain  Gain=0.1824
  Zq1 : Gain  Gain=0.1824
  id* : Outport
  iq* : Outport  Port=2
  tag scope: id_ref2=global, iq_ref2=global
  wires:
  Zd/1 -> Sum3/1
  Zq1/1 -> Sum3/2
  Zd1/1 -> Sum1/2
  Zq/1 -> Sum1/1
  Sum3/1 -> Divide/1
  Zd^2+Zq^2/1 -> Divide/2, Divide1/1, Scope24/1
  Sum1/1 -> Divide1/2
  evd/1 -> Zd/1, Zq/1
  evq/1 -> Zd1/1, Zq1/1
  Divide1/1 -> iq*/1, [iq_ref2]
  Divide/1 -> id*/1, [id_ref2]

== system parametrefarkli/Inverter Control1/Frequency Reference Generator ==
  note: theta
  Constant : Constant  Value=2*pi
  Integrator : Integrator  ExternalReset=rising
  Relational Operator : RelationalOperator  OutDataTypeStr=boolean  RndMeth=Nearest
  "f* " : Constant  Value=50
  w* : Gain  Gain=2*pi
  theta* : Outport
  wires:
  "f* "/1 -> w*/1
  w*/1 -> Integrator/1
  Relational Operator/1 -> Integrator/2
  Constant/1 -> Relational Operator/2
  Integrator/1 -> Relational Operator/1, theta*/1

== system parametrefarkli/Inverter Control1/Iabc  - idq ==
  Iabc : Inport
  theta : Inport  Port=2
  Demux : Demux  Outputs=2
  abc  - alfa/beta : Subsystem
  alfa/beta - dq : Subsystem
  iq : Outport
  id : Outport  Port=2
  tag scope: id2=global, iq2=global
  wires:
  theta/1 -> alfa/beta - dq/2(theta)
  Iabc/1 -> abc  - alfa/beta/1(abc)
  abc  - alfa/beta/1(alfa/beta) -> alfa/beta - dq/1(alfa/beta)
  alfa/beta - dq/1(d/q) -> Demux/1
  Demux/1 -> id/1, [id2]
  Demux/2 -> iq/1, [iq2]

== system parametrefarkli/Inverter Control1/PI id ==
  e : Inport
  Gain1 : Gain  Gain=50
  Gain2 : Gain  Gain=500
  Integrator : Integrator
  Saturation : Saturate  UpperLimit=inf  LowerLimit=-inf
  Sum1 : Sum  Inputs=|++
  " " : Outport
  wires:
  Sum1/1 -> Saturation/1
  Integrator/1 -> Sum1/2
  Gain1/1 -> Sum1/1
  e/1 -> Gain2/1, Gain1/1
  Gain2/1 -> Integrator/1
  Saturation/1 -> " "/1

== system parametrefarkli/Inverter Control1/PI iq ==
  e : Inport
  Gain1 : Gain  Gain=50
  Gain2 : Gain  Gain=500
  Integrator : Integrator
  Saturation : Saturate  UpperLimit=inf  LowerLimit=-inf
  Sum1 : Sum  Inputs=|++
  " " : Outport
  wires:
  Saturation/1 -> " "/1
  Gain2/1 -> Integrator/1
  e/1 -> Gain1/1, Gain2/1
  Gain1/1 -> Sum1/1
  Integrator/1 -> Sum1/2
  Sum1/1 -> Saturation/1

== system parametrefarkli/Inverter Control1/PI vd ==
  e : Inport
  Gain1 : Gain  Gain=2
  Gain2 : Gain  Gain=20
  Integrator : Integrator
  Saturation : Saturate  UpperLimit=inf  LowerLimit=-inf
  Sum1 : Sum  Inputs=|++
  " " : Outport
  wires:
  Saturation/1 -> " "/1
  Gain2/1 -> Integrator/1
  e/1 -> Gain1/1, Gain2/1
  Gain1/1 -> Sum1/1
  Integrator/1 -> Sum1/2
  Sum1/1 -> Saturation/1

== system parametrefarkli/Inverter Control1/PI vq ==
  e : Inport
  Gain1 : Gain  Gain=2
  Gain2 : Gain  Gain=2
  Integrator : Integrator
  Saturation : Saturate  UpperLimit=inf  LowerLimit=-inf
  Sum1 : Sum  Inputs=|++
  " " : Outport
  wires:
  Sum1/1 -> Saturation/1
  Integrator/1 -> Sum1/2
  Gain1/1 -> Sum1/1
  e/1 -> Gain2/1, Gain1/1
  Gain2/1 -> Integrator/1
  Saturation/1 -> " "/1

== system parametrefarkli/Inverter Control1/PWM ==
  Uabc_ref : Inport
  Gain2 : Gain  Gain=2/1000
  PWM Generator : powerlib_extras/Control  Blocks/PWM Generator  GeneratorMode="3-arm  bridge (6 pulses)"  Fc=10000  Internal=off  mIndex=0.4  Freq=60  Phase=0
  S : Outport
  tag scope: m_index2=global, pulses2=global
  wires:
  PWM Generator/1 -> S/1, [pulses2]
  Uabc_ref/1 -> Gain2/1
  Gain2/1 -> PWM Generator/1, [m_index2]

== system parametrefarkli/Inverter Control1/Vabc  - vdq ==
  Vabc : Inport
  theta : Inport  Port=2
  Demux : Demux  Outputs=2
  abc  - alfa/beta : Subsystem
  alfa/beta - dq : Subsystem
  vq : Outport
  vd : Outport  Port=2
  tag scope: vd2=global, vq2=global
  wires:
  Demux/2 -> vq/1, [vq2]
  Demux/1 -> vd/1, [vd2]
  alfa/beta - dq/1(d/q) -> Demux/1
  abc  - alfa/beta/1(alfa/beta) -> alfa/beta - dq/1(alfa/beta)
  Vabc/1 -> abc  - alfa/beta/1(abc)
  theta/1 -> alfa/beta - dq/2(theta)

== system parametrefarkli/Inverter Control1/vdq - Vabc ==
  Ud/Uq : Inport
  theta : Inport  Port=2
  alfa/beta - abc : Subsystem
  d/q - alfa/beta : Subsystem
  Uabc_ref : Outport
  wires:
  d/q - alfa/beta/1(alfa/beta) -> alfa/beta - abc/1(alfa/beta)
  Ud/Uq/1 -> d/q - alfa/beta/1(d/q)
  alfa/beta - abc/1(abc) -> Uabc_ref/1
  theta/1 -> d/q - alfa/beta/2(tita)

== system parametrefarkli/Inverter Control2/ Voltage Reference Generator ==
  Mux4 : Mux  Inputs=3
  Phase A reference : Sin  Amplitude=400*sqrt(2)/sqrt(3)  Frequency=2*pi*50  SampleTime=0
  Phase B reference : Sin  Amplitude=400*sqrt(2)/sqrt(3)  Frequency=2*pi*50  Phase=-2*pi/3  SampleTime=0
  Phase C reference : Sin  Amplitude=400*sqrt(2)/sqrt(3)  Frequency=2*pi*50  Phase=2*pi/3  SampleTime=0
  Product : Product  RndMeth=Zero
  Ramp : simulink/Sources/Ramp  slope=1/0.3  start=0  X0=0
  Saturation : Saturate  UpperLimit=1  LowerLimit=0
  Vabc* : Outport
  tag scope: Vabc_ref3=global
  wires:
  Phase B reference/1 -> Mux4/2
  Phase A reference/1 -> Mux4/1
  Phase C reference/1 -> Mux4/3
  Ramp/1 -> Saturation/1
  Saturation/1 -> Product/2
  Mux4/1 -> Vabc*/1, [Vabc_ref3]

== system parametrefarkli/Inverter Control2/Cross Terms ==
  id* : Inport
  iq* : Inport  Port=2
  Gain1 : Gain  Gain=-2*pi*50*3e-3
  Gain2 : Gain  Gain=2*pi*50*3e-3
  " q" : Outport
  " d" : Outport  Port=2
  wires:
  id*/1 -> Gain1/1
  iq*/1 -> Gain2/1
  Gain1/1 -> " d"/1
  Gain2/1 -> " q"/1
